simulink model "exp05p03"  (R2021a)
settings: Solver=VariableStepAuto  StartTime=0.0  StopTime=10.0  RelTol=1e-3
libraries: spsIGBTDiodeLib x4, spsTriangleGeneratorLib x2, spsCurrentMeasurementLib x1, spsDCVoltageSourceLib x1, spsSeriesRLCBranchLib x1, spsVoltageMeasurementLib x1, spspowerguiLib x1
settings Model: Creator=User  LastModifiedBy=User

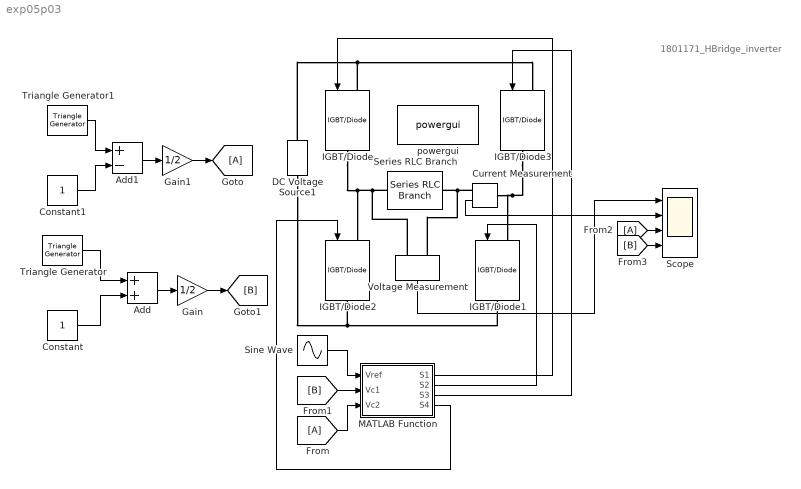
== system exp05p03 ==
  note: 1801171_HBridge_inverter
  Add : Sum
  Add1 : Sum  Inputs=+-
  Constant : Constant
  Constant1 : Constant
  Current Measurement : spsCurrentMeasurementLib/Current Measurement  PhasorSimulation=off  OutputType=Complex  PSBequivalent=0
  DC Voltage Source1 : spsDCVoltageSourceLib/DC Voltage Source  Amplitude=100  Measurements=None
  Gain : Gain  Gain=1/2
  Gain1 : Gain  Gain=1/2
  IGBT/Diode{,1..3} (4 alike) : spsIGBTDiodeLib/IGBT//Diode  Ron=1e-3  Rs=1e5  Cs=inf  Measurements=off
  MATLAB Function : MATLAB Function  TreatAsAtomicUnit=on
  Scope : Scope  NumInputPorts=4
  Series RLC Branch : spsSeriesRLCBranchLib/Series RLC Branch  LConnTagsString=__new0  RConnTagsString=__new0  BranchType=RL  Resistance=10  Inductance=1e-3  SetiL0=off  InitialCurrent=0  Capacitance=1e-6  Setx0=off  InitialVoltage=0  Measurements=None
  Sine Wave : Sin  SampleTime=0
  Triangle Generator : spsTriangleGeneratorLib/Triangle Generator  Freq=500  Phase=0  Ts=0
  Triangle Generator1 : spsTriangleGeneratorLib/Triangle Generator  Freq=500  Phase=0  Ts=0
  Voltage Measurement : spsVoltageMeasurementLib/Voltage Measurement  PhasorSimulation=off  OutputType=Complex  PSBequivalent=0
  powergui : spspowerguiLib/powergui  Priority=1  SimulationMode=Discrete  SampleTime=50e-6  frequency=60  Iterations=50  frequencyindice=0  Pbase=100e6  ErrMax=1e-4  UnitsV=kV  UnitsW=MW  buscounter=0  FunctionMessages=off  echomessages=off  EnableUseOfTLC=off  CurrentSourceSwitches=off  DisableSnubberDevices=off  DisableRonSwitches=off  DisableVfSwitches=off  DisplayEquations=off  AutomaticDiscreteSolvers=off  SolverType=Tustin/Backward Euler (TBE)  Interpol=off  ExternalGateDelay=off  methode=off  Ts=100  x0status=blocks  SPID=on  SwTol=0  HookPort=off  NonlinearTolerance=1e-4  nMaxIteration=100  ContinueOnMaxIteration=off  RestoreLinks=warning  ResistiveCurrentMeasurement=off  Frange=[0:2:500]  Ylog=off  Xlog=on  ShowGrid=off  save=off  variable=ZData  structure=0  ZoomFFT=off  StartTime=0.0  cycles=1  DisplayStyle=1  fundamental=60  FreqAxis=off  MaxFrequency=1000  frequencyindicesteady=1  RmsSteady=1  display=off
  wires:
  MATLAB Function/3(S3) -> IGBT/Diode3/1
  MATLAB Function/2(S2) -> IGBT/Diode1/1
  Current Measurement/1 -> Scope/2
  MATLAB Function/4(S4) -> IGBT/Diode2/1
  Voltage Measurement/1 -> Scope/1
  MATLAB Function/1(S1) -> IGBT/Diode/1
  Add/1 -> Gain/1
  Constant/1 -> Add/2
  Triangle Generator/1 -> Add/1
  Sine Wave/1 -> MATLAB Function/1(Vref)
  Triangle Generator1/1 -> Add1/1
  Constant1/1 -> Add1/2
  Add1/1 -> Gain1/1
  Gain1/1 -> [A]
  [A] -> MATLAB Function/3(Vc2)
  Gain/1 -> [B]
  [B] -> MATLAB Function/2(Vc1)
  [A] -> Scope/3
  [B] -> Scope/4
  connections:
  IGBT/Diode/RConn1 -- Series RLC Branch/RConn1 -- Voltage Measurement/LConn2 -- IGBT/Diode2/LConn1
  Series RLC Branch/LConn1 -- Voltage Measurement/LConn1 -- Current Measurement/RConn1
  DC Voltage Source1/RConn1 -- IGBT/Diode3/LConn1 -- IGBT/Diode/LConn1
  IGBT/Diode2/RConn1 -- IGBT/Diode1/RConn1 -- DC Voltage Source1/LConn1
  IGBT/Diode3/RConn1 -- IGBT/Diode1/LConn1 -- Current Measurement/LConn1

== matlab function exp05p03/MATLAB Function ==
  data: Vref input; S1 output; S2 output; S3 output; S4 output; Vc1 input; Vc2 input
function [S1,S2,S3,S4] = fcn(Vref,Vc1,Vc2)
%code_gen
if Vref>0
    if Vref>Vc1
    S1=1;
    S2=1;
    S3=0;
    S4=0;
    else
    S1=0;
    S2=0;
    S3=1;
    S4=1;
    end
else Vref<0
    if Vref<Vc2
    S1=0;
    S2=0;
    else
    S3=1;
    S4=1;
    end
end
end
